simulink model "Immersion_Invariance_Observer"  (R2020b)
settings: Solver=FixedStepAuto  StartTime=0.0  StopTime=10.0  FixedStep=DT  RelTol=1e-3
values from neighbouring files (symbols this model uses):
  gamma = (M_a(Omega_r_star + d_Omega_r, vx0, 0)         - M_a(Omega_r_star, vx0, 0)) / d_Omega_r    [eq_region2.m]    (also in eq_region3_cont.m = (M_a(Omega_r_star + d_Omega_r, vx0, theta_star)         - M_; run_Top_Model.m = 500)
  phi_0 = 0    [run_Top_Model.m]
  R = 63    [run_Top_Model.m]
  tp = turbine_params_5MW()    [baseline_design.m]    (also in run_Top_Model.m)
undefined symbols (not defined in the file or in its folder): A_pitch, B_pitch, C_pitch, II_vx0, ini_pitch, L_kal_pitch
libraries: simulink x1
settings Model: Creator=lpwoolcock  LastModifiedBy=lpwoolcock

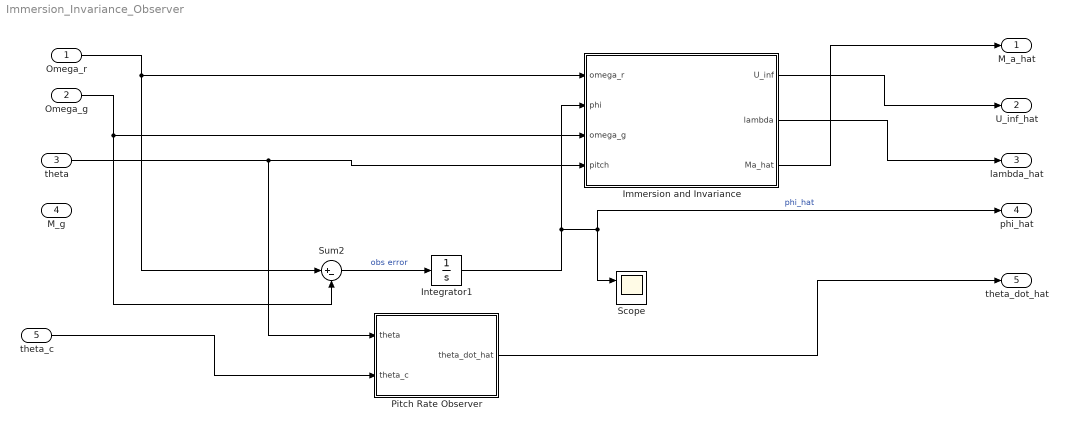
== system Immersion_Invariance_Observer ==
  Omega_r : Inport
  Omega_g : Inport  Port=2
  theta : Inport  Port=3
  M_g : Inport  Port=4
  theta_c : Inport  Port=5
  Immersion and Invariance : Subsystem  TreatAsAtomicUnit=on
  Integrator1 : Integrator  InitialCondition=phi_0
  Pitch Rate Observer : Subsystem  TreatAsAtomicUnit=on
  Scope : Scope  NumInputPorts=2
  Sum2 : Sum  Inputs=|+-
  M_a_hat : Outport
  U_inf_hat : Outport  Port=2
  lambda_hat : Outport  Port=3
  phi_hat : Outport  Port=4
  theta_dot_hat : Outport  Port=5
  wires:
  Sum2/1 -> Integrator1/1  "obs error"
  theta/1 -> Pitch Rate Observer/1(theta), Immersion and Invariance/4(pitch)
  Integrator1/1 -> Scope/1, phi_hat/1, Immersion and Invariance/2(phi)  "phi_hat"
  Omega_r/1 -> Immersion and Invariance/1(omega_r), Sum2/1
  Omega_g/1 -> Immersion and Invariance/3(omega_g), Sum2/2
  Immersion and Invariance/1(U_inf) -> U_inf_hat/1
  Immersion and Invariance/2(lambda) -> lambda_hat/1
  Immersion and Invariance/3(Ma_hat) -> M_a_hat/1
  theta_c/1 -> Pitch Rate Observer/2(theta_c)
  Pitch Rate Observer/1(theta_dot_hat) -> theta_dot_hat/1

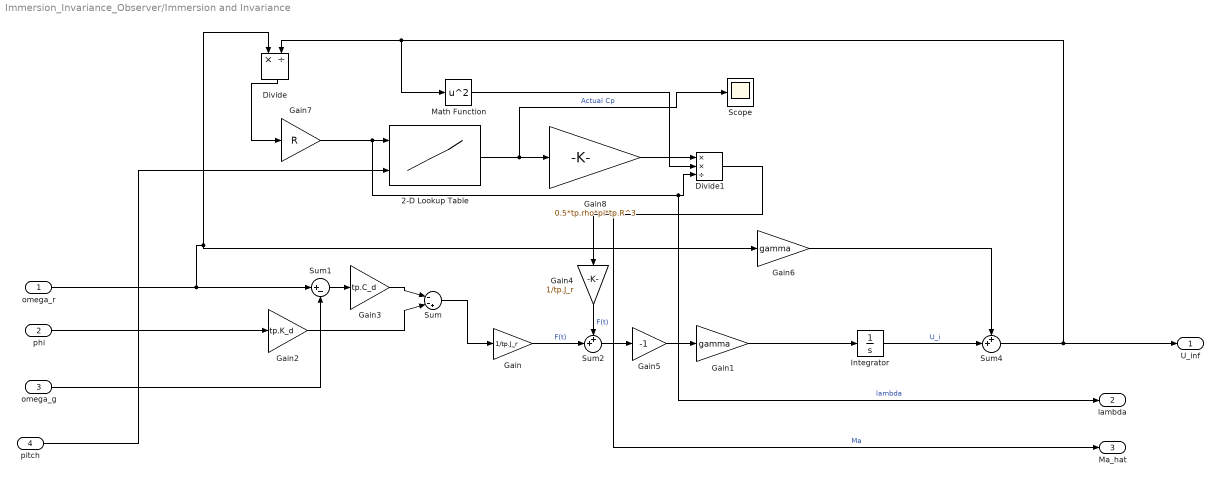
== system Immersion_Invariance_Observer/Immersion and Invariance ==
  omega_r : Inport
  phi : Inport  Port=2
  omega_g : Inport  Port=3
  pitch : Inport  Port=4
  2-D Lookup Table : Lookup_n-D  BreakpointsForDimension1=tp.lambda_bp  BreakpointsForDimension2=tp.theta_bp  Table=tp.C_p  InterpMethod=Cubic spline  ExtrapMethod=Cubic spline  InternalRulePriority=Speed  RndMeth=Simplest  InputSameDT=on
      settings: InputPortMap=u0,u1
  Divide : Product  Inputs=*/
  Divide1 : Product  Inputs=**/
  Gain : Gain  Gain=1/tp.J_r
  Gain1 : Gain  Gain=gamma
  Gain2 : Gain  Gain=tp.K_d
  Gain3 : Gain  Gain=tp.C_d
  Gain4 : Gain  Gain=1/tp.J_r
  Gain5 : Gain  Gain=-1
  Gain6 : Gain  Gain=gamma
  Gain7 : Gain  Gain=R
  Gain8 : Gain  Gain=0.5*tp.rho*pi*tp.R^3
  Integrator : Integrator  InitialCondition=II_vx0
  Math Function : Math  Operator=square  SaturateOnIntegerOverflow=on
  Scope : Scope
  Sum : Sum  Inputs=|--+
  Sum1 : Sum  Inputs=|+-
  Sum2 : Sum  Inputs=++|
  Sum4 : Sum  Inputs=++|
  U_inf : Outport
  lambda : Outport  Port=2
  Ma_hat : Outport  Port=3
  wires:
  phi/1 -> Gain2/1
  Gain2/1 -> Sum/2
  omega_g/1 -> Sum1/2
  Sum1/1 -> Gain3/1
  Gain3/1 -> Sum/1
  Sum/1 -> Gain/1
  omega_r/1 -> Sum1/1, Gain6/1, Divide/1
  Gain/1 -> Sum2/2  "F(t)"
  Gain4/1 -> Sum2/1  "F(t)"
  Sum2/1 -> Gain5/1
  Gain5/1 -> Gain1/1
  Integrator/1 -> Sum4/2  "U_i"
  Gain1/1 -> Integrator/1
  Gain6/1 -> Sum4/1
  pitch/1 -> 2-D Lookup Table/2
  Gain7/1 -> lambda/1, Divide1/3, 2-D Lookup Table/1  "lambda"
  Divide/1 -> Gain7/1
  Gain8/1 -> Divide1/1
  Divide1/1 -> Ma_hat/1, Gain4/1  "Ma"
  Math Function/1 -> Divide1/2
  2-D Lookup Table/1 -> Scope/1, Gain8/1  "Actual Cp"
  Sum4/1 -> Math Function/1, Divide/2, U_inf/1

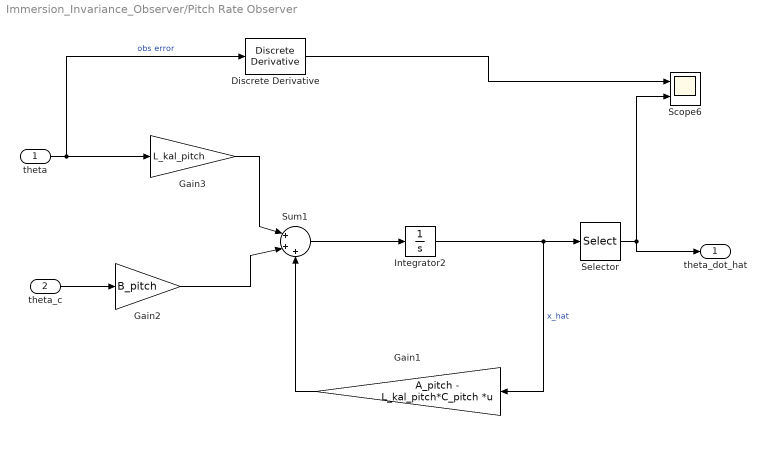
== system Immersion_Invariance_Observer/Pitch Rate Observer ==
  theta : Inport
  theta_c : Inport  Port=2
  Discrete Derivative : simulink/Discrete/Discrete Derivative  gainval=1.0  ICPrevScaledInput=0.0  OutMin=[]  OutMax=[]  OutDataType=fixdt(1, 16)  OutScaling=2^-10  DoSatur=off
  Gain1 : Gain  Gain=A_pitch - L_kal_pitch*C_pitch  Multiplication=Matrix(K*u)
  Gain2 : Gain  Gain=B_pitch
  Gain3 : Gain  Gain=L_kal_pitch
  Integrator2 : Integrator  InitialCondition=ini_pitch
  Scope6 : Scope  NumInputPorts=2
  Selector : Selector  InputPortWidth=2  IndexOptions=Index vector (dialog)  Indices=[2]  OutputSizes=1
  Sum1 : Sum  Inputs=|+++
  theta_dot_hat : Outport
  wires:
  Sum1/1 -> Integrator2/1
  Gain2/1 -> Sum1/2
  Gain3/1 -> Sum1/1
  Integrator2/1 -> Selector/1, Gain1/1  "x_hat"
  theta/1 -> Discrete Derivative/1, Gain3/1  "obs error"
  Gain1/1 -> Sum1/3
  theta_c/1 -> Gain2/1
  Selector/1 -> Scope6/2, theta_dot_hat/1
  Discrete Derivative/1 -> Scope6/1
